simulink model "DrawDifferentialEquationWaveform"  (R2014a)
settings: Solver=ode45  StartTime=0.0  StopTime=10.0  RelTol=1e-3
settings Model: Creator=tri  LastModifiedBy=tri

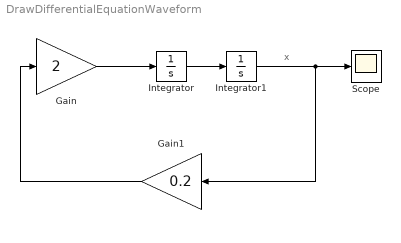
== system DrawDifferentialEquationWaveform ==
  note: x
  Gain : Gain  Gain=2
  Gain1 : Gain  Gain=0.2
  Integrator : Integrator
  Integrator1 : Integrator
  Scope : Scope
  wires:
  Integrator/1 -> Integrator1/1
  Gain/1 -> Integrator/1
  Integrator1/1 -> Scope/1, Gain1/1
  Gain1/1 -> Gain/1
